simulink model "ABS_Relay_Inf"  (Simulink 6.2)
settings: Solver=ode5  SolverMode=SingleTasking  StartTime=0.0  StopTime=400  FixedStep=0.01  RelTol=1e-3  AbsTol=1e-6
undefined symbols (not defined in the file): ABSPositionScale, ABSPowerScale, ABSTemperatureScale, ABSVelocityScale, mex_baseaddress
libraries: simulink_extras x3, simulink x2
settings Model: Creator=jims  LastModifiedBy=Administrator  ExtModeTrigDuration=40000
settings ConfigSet: SimulationMode=external
settings DataIOCC: ExternalInput=[]  InitialState=[]  LimitDataPoints=off  MaxDataPoints=5000  SaveOutput=off  SaveTime=off  SignalLoggingName=sigsOut
settings OptimizationCC: BlockReduction=off  BooleanDataType=off
settings DebuggingCC: IntegerOverflowMsg=none
settings HardwareCC: TargetEndianess=LittleEndian  TargetHWDeviceType=MATLAB Host
settings RTWCC: SystemTargetFile=rtwin.tlc  TemplateMakefile=rtwin.tmf  Description=Real-Time Windows Target  ProcessScript=rtwin_make_rtw_hook
settings RTWinTargetCC: TargetFcnLib=ansi_tfl_tmw.mat  GenFloatMathFcnCalls=ANSI_C  ModelReferenceCompliant=off  CCOptimize=on

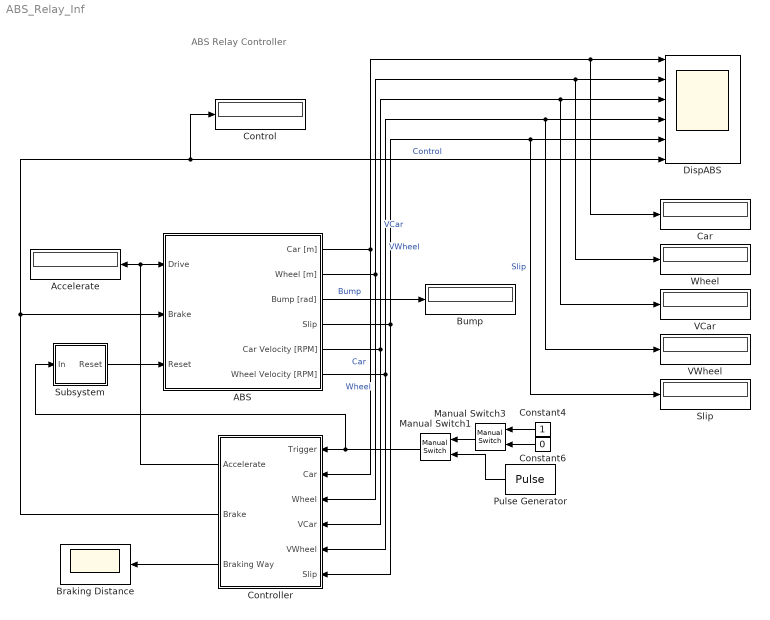
== system ABS_Relay_Inf ==
  note: ABS Relay Controller
  ABS : Subsystem  mask{BaseAddress=mex_baseaddress(-1,-1), T0=0.01}
      mask prompts: BaseAddress "Base Address"; T0 "Sample Time"
      mask Display: image(imread('abs.bmp'))
  Accelerate : Display
  Braking Distance : Scope
      settings: TimeRange=400  YMin=0  YMax=12  SaveName=ABSBrakingDistance  MaxDataPoints=40000
  Bump : Display
  Car : Display
  Constant4 : Constant  Orientation=left
  Constant6 : Constant  Orientation=left  Value=0
  Control : Display
  Controller : Subsystem  Orientation=left
  DispABS : Scope  NumInputPorts=6
      settings: TimeRange=400  YMin=0~0~0~0~-1.5~0  YMax=175~175~2500~2500~2~1  SaveName=ABSHistory  MaxDataPoints=40000
  Manual Switch1 : simulink/Signal Routing/Manual Switch  Orientation=left  sw=0  action=0
  Manual Switch3 : simulink/Signal Routing/Manual Switch  Orientation=left  sw=1  action=0
  Pulse Generator : DiscretePulseGenerator  Orientation=left  PulseType=Time based  Period=20  PulseWidth=90
  Slip : Display
  Subsystem : Subsystem
  VCar : Display
  VWheel : Display
  Wheel : Display
  wires:
  ABS/4(Slip) -> Slip/1, DispABS/5, Controller/6(Slip)  "Slip"
  ABS/6(Wheel Velocity [RPM]) -> VWheel/1, DispABS/4, Controller/5(VWheel)  "VWheel"
  ABS/2(Wheel [m]) -> Wheel/1, DispABS/2, Controller/3(Wheel)  "Wheel"
  ABS/1(Car [m]) -> Car/1, DispABS/1, Controller/2(Car)  "Car"
  Controller/3(Braking Way) -> Braking Distance/1
  Constant6/1 -> Manual Switch3/2
  Constant4/1 -> Manual Switch3/1
  Controller/2(Brake) -> Control/1, DispABS/6, ABS/2(Brake)  "Control"
  ABS/5(Car Velocity [RPM]) -> VCar/1, DispABS/3, Controller/4(VCar)  "VCar"
  ABS/3(Bump [rad]) -> Bump/1  "Bump"
  Controller/1(Accelerate) -> ABS/1(Drive), Accelerate/1
  Manual Switch3/1 -> Manual Switch1/1
  Pulse Generator/1 -> Manual Switch1/2
  Manual Switch1/1 -> Controller/1(Trigger), Subsystem/1(In)
  Subsystem/1(Reset) -> ABS/3(Reset)

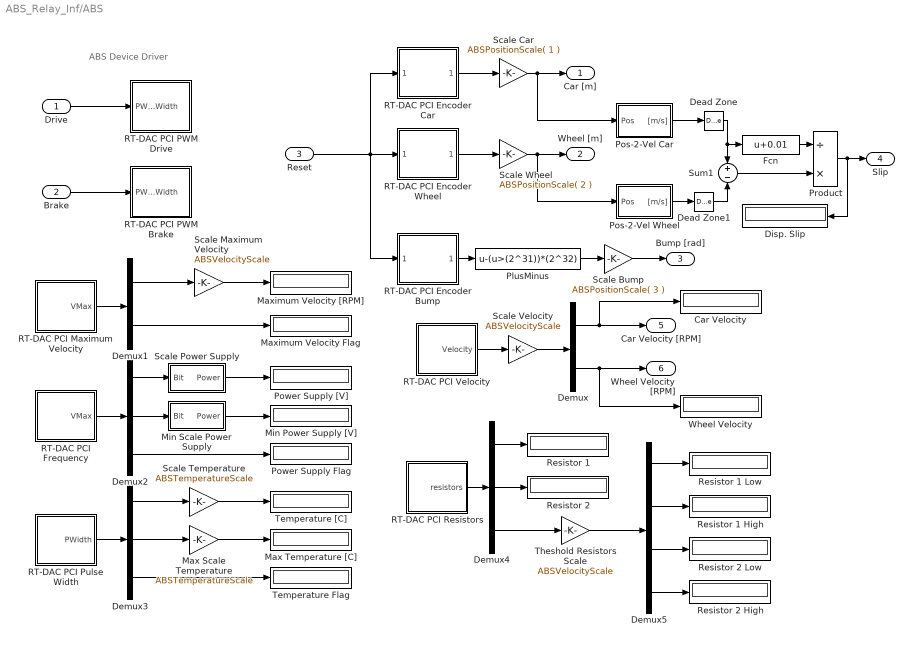
== system ABS_Relay_Inf/ABS ==
  note: ABS Device Driver
  Drive : Inport  Port=1  LatchInput=off
  Brake : Inport  Port=2  LatchInput=off
  Reset : Inport  Port=3  LatchInput=off
  Car Velocity : Display
  Dead Zone : DeadZone  LowerValue=-0.05  UpperValue=0.05  SaturateOnIntegerOverflow=on
  Dead Zone1 : DeadZone  LowerValue=-0.05  UpperValue=0.05  SaturateOnIntegerOverflow=on
  Demux : Demux  Outputs=2
  Demux1 : Demux  Outputs=2
  Demux2 : Demux  Outputs=3
  Demux3 : Demux  Outputs=3
  Demux4 : Demux  Outputs=[1 1 4]
  Demux5 : Demux
  Disp. Slip : Display
      settings: Format=bank
  Fcn : Fcn  Expr=u+0.01
  Max Scale Temperature : Gain  Gain=ABSTemperatureScale
  Max Temperature [C] : Display
  Maximum Velocity Flag : Display
  Maximum Velocity [RPM] : Display
  Min Power Supply [V] : Display
  Min Scale Power Supply : Subsystem
  PlusMinus : Fcn  Expr=u-(u>(2^31))*(2^32)
  Pos-2-Vel Car : Subsystem
  Pos-2-Vel Wheel : Subsystem
  Power Supply Flag : Display
  Power Supply [V] : Display
  Product : Product  Inputs=/*  SaturateOnIntegerOverflow=on  InputSameDT=on
  RT-DAC PCI Encoder Bump : Subsystem  mask(Incremental Encoders){BaseAddress=BaseAddress, ChannelIdx=2, T0=T0}
      mask prompts: BaseAddress "Base Address:"; ChannelIdx "Channel:"; T0 "Sample Time (sec):"
      mask help: RT-DAC PCI Device Driver
      mask Help: Set up each field for your specific hardware configuration.
      mask StyleString: edit,popup(0|1|2|3),edit
      mask Display: plot(0,0,100,100,[90,80,80,11,11],[90,90,20,20,80],[11,80],[80,80],[80,80],[20,14],[80,85,85,80],[45,45,66,66],[45,45,74,74],[20,13,13,20],[15,27,27,15,15],[75,75,26,26,75],[33,48,48,33,33],[75,75,55,55,75],[55,55,71,71,55],[55,75,75,55,55],[33,41,41,33,33],[50,50,27,27,50],[48,56,56,48,48],[50,50,27,27,50],[62,70,70,62,62],[50,50,27,27,50])
  RT-DAC PCI Encoder Car : Subsystem  mask(Incremental Encoders){BaseAddress=BaseAddress, ChannelIdx=0, T0=T0}
      mask prompts: BaseAddress "Base Address:"; ChannelIdx "Channel:"; T0 "Sample Time (sec):"
      mask help: RT-DAC PCI Device Driver
      mask Help: Set up each field for your specific hardware configuration.
      mask StyleString: edit,popup(0|1|2|3),edit
      mask Display: plot(0,0,100,100,[90,80,80,11,11],[90,90,20,20,80],[11,80],[80,80],[80,80],[20,14],[80,85,85,80],[45,45,66,66],[45,45,74,74],[20,13,13,20],[15,27,27,15,15],[75,75,26,26,75],[33,48,48,33,33],[75,75,55,55,75],[55,55,71,71,55],[55,75,75,55,55],[33,41,41,33,33],[50,50,27,27,50],[48,56,56,48,48],[50,50,27,27,50],[62,70,70,62,62],[50,50,27,27,50])
  RT-DAC PCI Encoder Wheel : Subsystem  mask(Incremental Encoders){BaseAddress=BaseAddress, ChannelIdx=1, T0=T0}
      mask prompts: BaseAddress "Base Address:"; ChannelIdx "Channel:"; T0 "Sample Time (sec):"
      mask help: RT-DAC PCI Device Driver
      mask Help: Set up each field for your specific hardware configuration.
      mask StyleString: edit,popup(0|1|2|3),edit
      mask Display: plot(0,0,100,100,[90,80,80,11,11],[90,90,20,20,80],[11,80],[80,80],[80,80],[20,14],[80,85,85,80],[45,45,66,66],[45,45,74,74],[20,13,13,20],[15,27,27,15,15],[75,75,26,26,75],[33,48,48,33,33],[75,75,55,55,75],[55,55,71,71,55],[55,75,75,55,55],[33,41,41,33,33],[50,50,27,27,50],[48,56,56,48,48],[50,50,27,27,50],[62,70,70,62,62],[50,50,27,27,50])
  RT-DAC PCI Frequency : Subsystem  mask(Incremental Encoders){BaseAddress=BaseAddress, T0=T0}
      mask prompts: BaseAddress "Base Address:"; T0 "Sample Time (sec):"
      mask help: RT-DAC PCI Device Driver
      mask Help: Set up each field for your specific hardware configuration.
      mask Display: plot(0,0,100,100,[90,80,80,11,11],[90,90,20,20,80],[11,80],[80,80],[80,80],[20,14],[80,85,85,80],[45,45,66,66],[45,45,74,74],[20,13,13,20],[15,27,27,15,15],[75,75,26,26,75],[33,48,48,33,33],[75,75,55,55,75],[55,55,71,71,55],[55,75,75,55,55],[33,41,41,33,33],[50,50,27,27,50],[48,56,56,48,48],[50,50,27,27,50],[62,70,70,62,62],[50,50,27,27,50])
  RT-DAC PCI Maximum Velocity : Subsystem  mask(Incremental Encoders){BaseAddress=BaseAddress, T0=T0}
      mask prompts: BaseAddress "Base Address:"; T0 "Sample Time (sec):"
      mask help: RT-DAC PCI Device Driver
      mask Help: Set up each field for your specific hardware configuration.
      mask Display: plot(0,0,100,100,[90,80,80,11,11],[90,90,20,20,80],[11,80],[80,80],[80,80],[20,14],[80,85,85,80],[45,45,66,66],[45,45,74,74],[20,13,13,20],[15,27,27,15,15],[75,75,26,26,75],[33,48,48,33,33],[75,75,55,55,75],[55,55,71,71,55],[55,75,75,55,55],[33,41,41,33,33],[50,50,27,27,50],[48,56,56,48,48],[50,50,27,27,50],[62,70,70,62,62],[50,50,27,27,50])
  RT-DAC PCI PWM Brake : Subsystem  mask(PWM Module){BaseAddress=BaseAddress, ChanIdx=1, ChanMode=12 Bit, ChanPresc=60, SetOutputsFlag=on, SetOutputsValue=0, T0=T0}
      mask prompts: BaseAddress "IO Base Address:"; ChanIdx "Channel:"; ChanMode "Channel Mode:"; ChanPresc "Channel Prescaler:"; SetOutputsFlag "Set Outputs At Termination"; SetOutputsValue "Termination Outputs:"; T0 "Sample Time (sec):"
      mask help: RT-DAC PCI Device Driver
      mask Help: Set up each field for your specific hardware configuration.
      mask StyleString: edit,popup(0|1|2|3),popup(8 Bit|12 Bit),edit,checkbox,edit,edit
      mask Display: plot(0,0,100,100,[90,80,80,11,11],[90,90,20,20,80],[11,80],[80,80],[80,80],[20,14],[80,85,85,80],[45,45,66,66],[45,45,74,74],[20,13,13,20],[15,27,27,15,15],[75,75,26,26,75],[33,48,48,33,33],[75,75,55,55,75],[55,55,71,71,55],[55,75,75,55,55],[33,41,41,33,33],[50,50,27,27,50],[48,56,56,48,48],[50,50,27,27,50],[62,70,70,62,62],[50,50,27,27,50])
  RT-DAC PCI PWM Drive : Subsystem  mask(PWM Module){BaseAddress=BaseAddress, ChanIdx=0, ChanMode=12 Bit, ChanPresc=60, SetOutputsFlag=on, SetOutputsValue=0, T0=T0}
      mask prompts: BaseAddress "IO Base Address:"; ChanIdx "Channel:"; ChanMode "Channel Mode:"; ChanPresc "Channel Prescaler:"; SetOutputsFlag "Set Outputs At Termination"; SetOutputsValue "Termination Outputs:"; T0 "Sample Time (sec):"
      mask help: RT-DAC PCI Device Driver
      mask Help: Set up each field for your specific hardware configuration.
      mask StyleString: edit,popup(0|1|2|3),popup(8 Bit|12 Bit),edit,checkbox,edit,edit
      mask Display: plot(0,0,100,100,[90,80,80,11,11],[90,90,20,20,80],[11,80],[80,80],[80,80],[20,14],[80,85,85,80],[45,45,66,66],[45,45,74,74],[20,13,13,20],[15,27,27,15,15],[75,75,26,26,75],[33,48,48,33,33],[75,75,55,55,75],[55,55,71,71,55],[55,75,75,55,55],[33,41,41,33,33],[50,50,27,27,50],[48,56,56,48,48],[50,50,27,27,50],[62,70,70,62,62],[50,50,27,27,50])
  RT-DAC PCI Pulse Width : Subsystem  mask(Incremental Encoders){BaseAddress=BaseAddress, T0=T0}
      mask prompts: BaseAddress "Base Address:"; T0 "Sample Time (sec):"
      mask help: RT-DAC PCI Device Driver
      mask Help: Set up each field for your specific hardware configuration.
      mask Display: plot(0,0,100,100,[90,80,80,11,11],[90,90,20,20,80],[11,80],[80,80],[80,80],[20,14],[80,85,85,80],[45,45,66,66],[45,45,74,74],[20,13,13,20],[15,27,27,15,15],[75,75,26,26,75],[33,48,48,33,33],[75,75,55,55,75],[55,55,71,71,55],[55,75,75,55,55],[33,41,41,33,33],[50,50,27,27,50],[48,56,56,48,48],[50,50,27,27,50],[62,70,70,62,62],[50,50,27,27,50])
  RT-DAC PCI Resistors : Subsystem  mask(Incremental Encoders){BaseAddress=BaseAddress, T0=T0}
      mask prompts: BaseAddress "Base Address:"; T0 "Sample Time (sec):"
      mask help: RT-DAC PCI Device Driver
      mask Help: Set up each field for your specific hardware configuration.
      mask Display: plot(0,0,100,100,[90,80,80,11,11],[90,90,20,20,80],[11,80],[80,80],[80,80],[20,14],[80,85,85,80],[45,45,66,66],[45,45,74,74],[20,13,13,20],[15,27,27,15,15],[75,75,26,26,75],[33,48,48,33,33],[75,75,55,55,75],[55,55,71,71,55],[55,75,75,55,55],[33,41,41,33,33],[50,50,27,27,50],[48,56,56,48,48],[50,50,27,27,50],[62,70,70,62,62],[50,50,27,27,50])
  RT-DAC PCI Velocity : Subsystem  mask(Incremental Encoders){BaseAddress=BaseAddress, T0=T0}
      mask prompts: BaseAddress "Base Address:"; T0 "Sample Time (sec):"
      mask help: RT-DAC PCI Device Driver
      mask Help: Set up each field for your specific hardware configuration.
      mask Display: plot(0,0,100,100,[90,80,80,11,11],[90,90,20,20,80],[11,80],[80,80],[80,80],[20,14],[80,85,85,80],[45,45,66,66],[45,45,74,74],[20,13,13,20],[15,27,27,15,15],[75,75,26,26,75],[33,48,48,33,33],[75,75,55,55,75],[55,55,71,71,55],[55,75,75,55,55],[33,41,41,33,33],[50,50,27,27,50],[48,56,56,48,48],[50,50,27,27,50],[62,70,70,62,62],[50,50,27,27,50])
  Resistor 1 : Display
  Resistor 1 High : Display
  Resistor 1 Low : Display
  Resistor 2 : Display
  Resistor 2 High : Display
  Resistor 2 Low : Display
  Scale Bump : Gain  Gain=ABSPositionScale( 3 )
  Scale Car : Gain  Gain=ABSPositionScale( 1 )
  Scale Maximum Velocity : Gain  Gain=ABSVelocityScale
  Scale Velocity : Gain  Gain=ABSVelocityScale
  Scale Wheel : Gain  Gain=ABSPositionScale( 2 )
  Scale Power Supply : Subsystem
  Scale Temperature : Gain  Gain=ABSTemperatureScale
  Sum1 : Sum  Inputs=+-  SaturateOnIntegerOverflow=on  InputSameDT=on
  Temperature Flag : Display
  Temperature [C] : Display
  Theshold Resistors Scale : Gain  Gain=ABSVelocityScale
  Wheel Velocity : Display
  Car [m] : Outport
  Wheel [m] : Outport  Port=2
  Bump [rad] : Outport  Port=3
  Slip : Outport  Port=4
  Car Velocity [RPM] : Outport  Port=5
  Wheel Velocity [RPM] : Outport  Port=6
  wires:
  Dead Zone1/1 -> Sum1/2
  Dead Zone/1 -> Fcn/1, Sum1/1
  Pos-2-Vel Car/1("[m/s]") -> Dead Zone/1
  Pos-2-Vel Wheel/1("[m/s]") -> Dead Zone1/1
  Product/1 -> Disp. Slip/1, Slip/1
  Fcn/1 -> Product/1
  Sum1/1 -> Product/2
  Demux5/4 -> Resistor 2 High/1
  Demux5/3 -> Resistor 2 Low/1
  Demux5/2 -> Resistor 1 High/1
  Demux5/1 -> Resistor 1 Low/1
  Theshold Resistors Scale/1 -> Demux5/1
  Demux4/3 -> Theshold Resistors Scale/1
  Demux4/2 -> Resistor 2/1
  Demux4/1 -> Resistor 1/1
  RT-DAC PCI Resistors/1(resistors) -> Demux4/1
  Demux3/3 -> Temperature Flag/1
  Demux3/2 -> Max Scale Temperature/1
  Max Scale Temperature/1 -> Max Temperature [C]/1
  Demux2/3 -> Power Supply Flag/1
  Min Scale Power Supply/1(Power) -> Min Power Supply [V]/1
  Demux2/2 -> Min Scale Power Supply/1(Bit)
  Reset/1 -> RT-DAC PCI Encoder Bump/1(Reset), RT-DAC PCI Encoder Car/1(Reset), RT-DAC PCI Encoder Wheel/1(Reset)
  Demux3/1 -> Scale Temperature/1
  RT-DAC PCI Pulse Width/1(PWidth) -> Demux3/1
  Demux2/1 -> Scale Power Supply/1(Bit)
  RT-DAC PCI Frequency/1(VMax) -> Demux2/1
  Demux1/2 -> Maximum Velocity Flag/1
  Scale Maximum Velocity/1 -> Maximum Velocity [RPM]/1
  Demux1/1 -> Scale Maximum Velocity/1
  RT-DAC PCI Maximum Velocity/1(VMax) -> Demux1/1
  Demux/2 -> Wheel Velocity/1, Wheel Velocity [RPM]/1
  Demux/1 -> Car Velocity/1, Car Velocity [RPM]/1
  Brake/1 -> RT-DAC PCI PWM Brake/1(PWM Width)
  Drive/1 -> RT-DAC PCI PWM Drive/1(PWM Width)
  Scale Temperature/1 -> Temperature [C]/1
  Scale Power Supply/1(Power) -> Power Supply [V]/1
  Scale Velocity/1 -> Demux/1
  RT-DAC PCI Velocity/1(Velocity) -> Scale Velocity/1
  Scale Bump/1 -> Bump [rad]/1
  Scale Wheel/1 -> Pos-2-Vel Wheel/1(Pos), Wheel [m]/1
  Scale Car/1 -> Pos-2-Vel Car/1(Pos), Car [m]/1
  RT-DAC PCI Encoder Bump/1(Encoder Counter) -> PlusMinus/1
  RT-DAC PCI Encoder Wheel/1(Encoder Counter) -> Scale Wheel/1
  RT-DAC PCI Encoder Car/1(Encoder Counter) -> Scale Car/1
  PlusMinus/1 -> Scale Bump/1

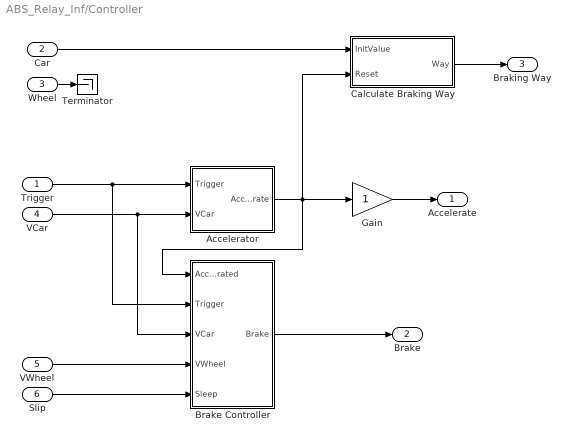
== system ABS_Relay_Inf/Controller ==
  Trigger : Inport  Port=1  LatchInput=off
  Car : Inport  Port=2  LatchInput=off
  Wheel : Inport  Port=3  LatchInput=off
  VCar : Inport  Port=4  LatchInput=off
  VWheel : Inport  Port=5  LatchInput=off
  Slip : Inport  Port=6  LatchInput=off
  Accelerator : Subsystem
  Brake Controller : Subsystem
  Calculate Braking Way : Subsystem
  Gain : Gain  SaturateOnIntegerOverflow=on
  Terminator : Terminator
  Accelerate : Outport
  Brake : Outport  Port=2
  Braking Way : Outport  Port=3
  wires:
  Gain/1 -> Accelerate/1
  Wheel/1 -> Terminator/1
  Brake Controller/1(Brake) -> Brake/1
  VWheel/1 -> Brake Controller/4(VWheel)
  Accelerator/1(Accelerate) -> Gain/1, Brake Controller/1(Accelerated), Calculate Braking Way/2(Reset)
  Slip/1 -> Brake Controller/5(Sleep)
  Car/1 -> Calculate Braking Way/1(InitValue)
  VCar/1 -> Accelerator/2(VCar), Brake Controller/3(VCar)
  Calculate Braking Way/1(Way) -> Braking Way/1
  Trigger/1 -> Brake Controller/2(Trigger), Accelerator/1(Trigger)

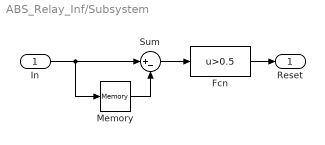
== system ABS_Relay_Inf/Subsystem ==
  In : Inport  Port=1  LatchInput=off
  Fcn : Fcn  Expr=u>0.5
  Memory : Memory
  Sum : Sum  Inputs=|+-  SaturateOnIntegerOverflow=on  InputSameDT=on
  Reset : Outport
  wires:
  Sum/1 -> Fcn/1
  In/1 -> Sum/1, Memory/1
  Fcn/1 -> Reset/1
  Memory/1 -> Sum/2

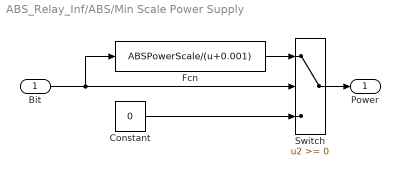
== system ABS_Relay_Inf/ABS/Min Scale Power Supply ==
  Bit : Inport  Port=1  LatchInput=off
  Constant : Constant  Value=0
  Fcn : Fcn  Expr=ABSPowerScale/(u+0.001)
  Switch : Switch  SaturateOnIntegerOverflow=on  InputSameDT=on
  Power : Outport
  wires:
  Bit/1 -> Switch/2, Fcn/1
  Switch/1 -> Power/1
  Fcn/1 -> Switch/1
  Constant/1 -> Switch/3

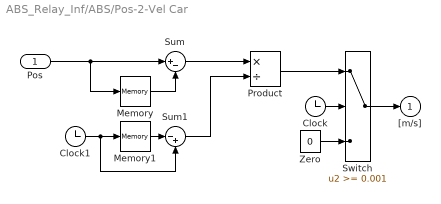
== system ABS_Relay_Inf/ABS/Pos-2-Vel Car ==
  Pos : Inport  Port=1  LatchInput=off
  Clock : Clock
      settings: Decimation=10
  Clock1 : Clock
      settings: Decimation=10
  Memory : Memory  InheritSampleTime=on
  Memory1 : Memory  InheritSampleTime=on
  Product : Product  Inputs=*/  SaturateOnIntegerOverflow=on  InputSameDT=on
  Sum : Sum  Inputs=|+-  SaturateOnIntegerOverflow=on  InputSameDT=on
  Sum1 : Sum  Inputs=|-+  SaturateOnIntegerOverflow=on  InputSameDT=on
  Switch : Switch  Threshold=0.001  SaturateOnIntegerOverflow=on  InputSameDT=on
  Zero : Constant  Value=0
  "[m/s]" : Outport  InitialOutput=0
  wires:
  Pos/1 -> Memory/1, Sum/1
  Memory/1 -> Sum/2
  Clock/1 -> Switch/2
  Switch/1 -> "[m/s]"/1
  Zero/1 -> Switch/3
  Product/1 -> Switch/1
  Sum/1 -> Product/1
  Clock1/1 -> Memory1/1, Sum1/2
  Memory1/1 -> Sum1/1
  Sum1/1 -> Product/2

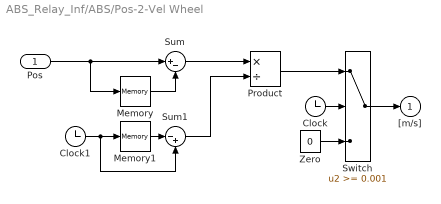
== system ABS_Relay_Inf/ABS/Pos-2-Vel Wheel ==
  Pos : Inport  Port=1  LatchInput=off
  Clock : Clock
      settings: Decimation=10
  Clock1 : Clock
      settings: Decimation=10
  Memory : Memory  InheritSampleTime=on
  Memory1 : Memory  InheritSampleTime=on
  Product : Product  Inputs=*/  SaturateOnIntegerOverflow=on  InputSameDT=on
  Sum : Sum  Inputs=|+-  SaturateOnIntegerOverflow=on  InputSameDT=on
  Sum1 : Sum  Inputs=|-+  SaturateOnIntegerOverflow=on  InputSameDT=on
  Switch : Switch  Threshold=0.001  SaturateOnIntegerOverflow=on  InputSameDT=on
  Zero : Constant  Value=0
  "[m/s]" : Outport  InitialOutput=0
  wires:
  Sum1/1 -> Product/2
  Memory1/1 -> Sum1/1
  Clock1/1 -> Sum1/2, Memory1/1
  Sum/1 -> Product/1
  Product/1 -> Switch/1
  Zero/1 -> Switch/3
  Switch/1 -> "[m/s]"/1
  Clock/1 -> Switch/2
  Memory/1 -> Sum/2
  Pos/1 -> Sum/1, Memory/1

== system ABS_Relay_Inf/ABS/RT-DAC PCI Encoder Bump ==
  Reset : Inport  Port=1  LatchInput=off
  RT-DAC PCI Encoder : S-Function  FunctionName=rtdacpci_abs_encoder  Parameters=BaseAddress, ChannelIdx, T0
  Encoder Counter : Outport  InitialOutput=0
  wires:
  RT-DAC PCI Encoder/1 -> Encoder Counter/1
  Reset/1 -> RT-DAC PCI Encoder/1

== system ABS_Relay_Inf/ABS/RT-DAC PCI Encoder Car ==
  Reset : Inport  Port=1  LatchInput=off
  RT-DAC PCI Encoder : S-Function  FunctionName=rtdacpci_abs_encoder  Parameters=BaseAddress, ChannelIdx, T0
  Encoder Counter : Outport  InitialOutput=0
  wires:
  RT-DAC PCI Encoder/1 -> Encoder Counter/1
  Reset/1 -> RT-DAC PCI Encoder/1

== system ABS_Relay_Inf/ABS/RT-DAC PCI Encoder Wheel ==
  Reset : Inport  Port=1  LatchInput=off
  RT-DAC PCI Encoder : S-Function  FunctionName=rtdacpci_abs_encoder  Parameters=BaseAddress, ChannelIdx, T0
  Encoder Counter : Outport  InitialOutput=0
  wires:
  Reset/1 -> RT-DAC PCI Encoder/1
  RT-DAC PCI Encoder/1 -> Encoder Counter/1

== system ABS_Relay_Inf/ABS/RT-DAC PCI Frequency ==
  RT-DAC PCI Frequency : S-Function  FunctionName=rtdacpci_abs_frequency  Parameters=BaseAddress, T0
  VMax : Outport  InitialOutput=0
  wires:
  RT-DAC PCI Frequency/1 -> VMax/1

== system ABS_Relay_Inf/ABS/RT-DAC PCI Maximum Velocity ==
  RT-DAC PCI VMax : S-Function  FunctionName=rtdacpci_abs_vmax  Parameters=BaseAddress, T0
  VMax : Outport  InitialOutput=0
  wires:
  RT-DAC PCI VMax/1 -> VMax/1

== system ABS_Relay_Inf/ABS/RT-DAC PCI PWM Brake ==
  PWM Width : Inport  Port=1  LatchInput=off
  "RT-DAC PCI PWM " : S-Function  FunctionName=rtdacpci_abs_pwm  Parameters=BaseAddress, ChanIdx, ChanMode, ChanPresc, SetOutputsFlag, SetOutputsValue, T0
  wires:
  PWM Width/1 -> "RT-DAC PCI PWM "/1

== system ABS_Relay_Inf/ABS/RT-DAC PCI PWM Drive ==
  PWM Width : Inport  Port=1  LatchInput=off
  "RT-DAC PCI PWM " : S-Function  FunctionName=rtdacpci_abs_pwm  Parameters=BaseAddress, ChanIdx, ChanMode, ChanPresc, SetOutputsFlag, SetOutputsValue, T0
  wires:
  PWM Width/1 -> "RT-DAC PCI PWM "/1

== system ABS_Relay_Inf/ABS/RT-DAC PCI Pulse Width ==
  RT-DAC PCI Pulse Width : S-Function  FunctionName=rtdacpci_abs_pulsewidth  Parameters=BaseAddress, T0
  PWidth : Outport  InitialOutput=0
  wires:
  RT-DAC PCI Pulse Width/1 -> PWidth/1

== system ABS_Relay_Inf/ABS/RT-DAC PCI Resistors ==
  RT-DAC PCI Resistors : S-Function  FunctionName=rtdacpci_abs_resistors  Parameters=BaseAddress, T0
  resistors : Outport  InitialOutput=0
  wires:
  RT-DAC PCI Resistors/1 -> resistors/1

== system ABS_Relay_Inf/ABS/RT-DAC PCI Velocity ==
  RT-DAC PCI Velocity : S-Function  FunctionName=rtdacpci_abs_velocity  Parameters=BaseAddress, T0
  Velocity : Outport  InitialOutput=0
  wires:
  RT-DAC PCI Velocity/1 -> Velocity/1

== system ABS_Relay_Inf/ABS/Scale Power Supply ==
  Bit : Inport  Port=1  LatchInput=off
  Constant : Constant  Value=0
  Fcn : Fcn  Expr=ABSPowerScale/(u+0.001)
  Switch : Switch  Threshold=0.5  SaturateOnIntegerOverflow=on  InputSameDT=on
  Power : Outport
  wires:
  Constant/1 -> Switch/3
  Fcn/1 -> Switch/1
  Switch/1 -> Power/1
  Bit/1 -> Fcn/1, Switch/2

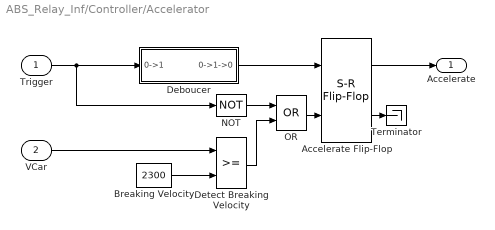
== system ABS_Relay_Inf/Controller/Accelerator ==
  Trigger : Inport  Port=1  LatchInput=off
  VCar : Inport  Port=2  LatchInput=off
  Accelerate Flip-Flop : simulink_extras/Flip Flops/S-R Flip-Flop  initial_condition=0
  Breaking Velocity : Constant  Value=2300
  Deboucer : Subsystem
  Detect Breaking Velocity : RelationalOperator  InputSameDT=on
  NOT : Logic  Operator=NOT
  OR : Logic  Operator=OR
  Terminator : Terminator
  Accelerate : Outport
  wires:
  Accelerate Flip-Flop/1 -> Accelerate/1
  VCar/1 -> Detect Breaking Velocity/1
  Trigger/1 -> NOT/1, Deboucer/1(0->1)
  Accelerate Flip-Flop/2 -> Terminator/1
  NOT/1 -> OR/1
  Detect Breaking Velocity/1 -> OR/2
  OR/1 -> Accelerate Flip-Flop/2
  Breaking Velocity/1 -> Detect Breaking Velocity/2
  Deboucer/1(0->1->0) -> Accelerate Flip-Flop/1

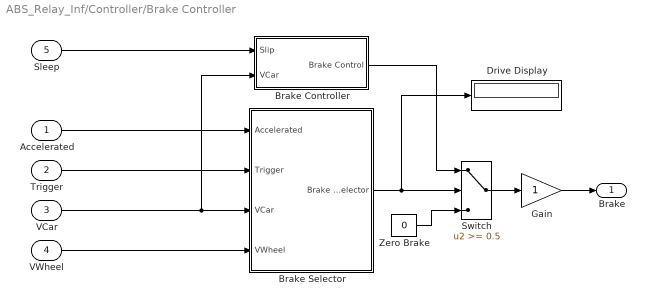
== system ABS_Relay_Inf/Controller/Brake Controller ==
  Accelerated : Inport  Port=1  LatchInput=off
  Trigger : Inport  Port=2  LatchInput=off
  VCar : Inport  Port=3  LatchInput=off
  VWheel : Inport  Port=4  LatchInput=off
  Sleep : Inport  Port=5  LatchInput=off
  Brake Controller : Subsystem
  Brake Selector : Subsystem
  Drive Display : Display
  Gain : Gain  SaturateOnIntegerOverflow=on
  Switch : Switch  Threshold=0.5  InputSameDT=on
  Zero Brake : Constant  Value=0
  Brake : Outport
  wires:
  Gain/1 -> Brake/1
  Brake Controller/1(Brake Control) -> Switch/1
  Sleep/1 -> Brake Controller/1(Slip)
  Zero Brake/1 -> Switch/3
  Brake Selector/1(Brake Selector) -> Drive Display/1, Switch/2
  Switch/1 -> Gain/1
  VWheel/1 -> Brake Selector/4(VWheel)
  VCar/1 -> Brake Controller/2(VCar), Brake Selector/3(VCar)
  Trigger/1 -> Brake Selector/2(Trigger)
  Accelerated/1 -> Brake Selector/1(Accelerated)

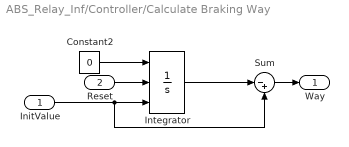
== system ABS_Relay_Inf/Controller/Calculate Braking Way ==
  InitValue : Inport  Port=1  LatchInput=off
  Reset : Inport  Port=2  LatchInput=off
  Constant2 : Constant  Value=0
  Integrator : Integrator  ExternalReset=level  InitialConditionSource=external
  Sum : Sum  Inputs=|-+  SaturateOnIntegerOverflow=on  InputSameDT=on
  Way : Outport
  wires:
  Sum/1 -> Way/1
  Reset/1 -> Integrator/2
  InitValue/1 -> Integrator/3, Sum/2
  Integrator/1 -> Sum/1
  Constant2/1 -> Integrator/1

== system ABS_Relay_Inf/Controller/Accelerator/Deboucer ==
  0->1 : Inport  Port=1  LatchInput=off
  AND : Logic
  Memory : Memory
  NOT : Logic  Operator=NOT
  0->1->0 : Outport
  wires:
  AND/1 -> 0->1->0/1
  0->1/1 -> Memory/1, AND/2
  Memory/1 -> NOT/1
  NOT/1 -> AND/1

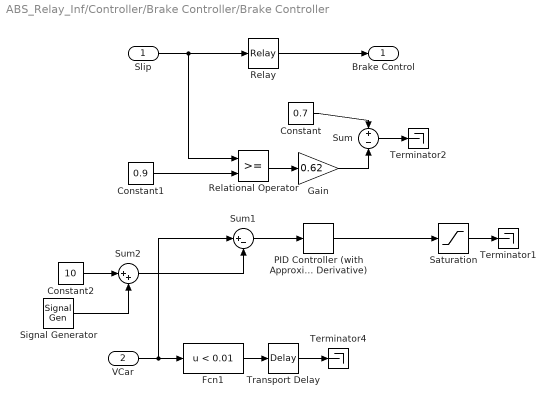
== system ABS_Relay_Inf/Controller/Brake Controller/Brake Controller ==
  Slip : Inport  Port=1  LatchInput=off
  VCar : Inport  Port=2  LatchInput=off
  Constant : Constant  Value=0.7
  Constant1 : Constant  Value=0.9
  Constant2 : Constant  Value=10
  Fcn1 : Fcn  Expr=u < 0.01
  Gain : Gain  Gain=0.62  SaturateOnIntegerOverflow=on
  PID Controller (with Approximate Derivative) : simulink_extras/Additional Linear/PID Controller (with Approximate Derivative)  P=0.2  I=0  D=0  N=100
  Relational Operator : RelationalOperator  InputSameDT=on
  Relay : Relay  OnSwitchValue=0.25  OffSwitchValue=0.1  OnOutputValue=0  OffOutputValue=1
  Saturation : Saturate  UpperLimit=0.7  LowerLimit=0
  Signal Generator : SignalGenerator  WaveForm=square  Amplitude=2  Frequency=0.03
  Sum : Sum  Inputs=+-  SaturateOnIntegerOverflow=on  InputSameDT=on
  Sum1 : Sum  Inputs=|+-  SaturateOnIntegerOverflow=on  InputSameDT=on
  Sum2 : Sum  Inputs=|++  SaturateOnIntegerOverflow=on  InputSameDT=on
  Terminator1 : Terminator
  Terminator2 : Terminator
  Terminator4 : Terminator
  Transport Delay : TransportDelay  DelayTime=0.5
  Brake Control : Outport
  wires:
  Slip/1 -> Relational Operator/1, Relay/1
  Fcn1/1 -> Transport Delay/1
  VCar/1 -> Fcn1/1, Sum1/1
  Relational Operator/1 -> Gain/1
  Constant1/1 -> Relational Operator/2
  Constant/1 -> Sum/1
  Gain/1 -> Sum/2
  Sum1/1 -> PID Controller (with Approximate Derivative)/1
  PID Controller (with Approximate Derivative)/1 -> Saturation/1
  Sum2/1 -> Sum1/2
  Constant2/1 -> Sum2/1
  Signal Generator/1 -> Sum2/2
  Relay/1 -> Brake Control/1
  Sum/1 -> Terminator2/1
  Saturation/1 -> Terminator1/1
  Transport Delay/1 -> Terminator4/1

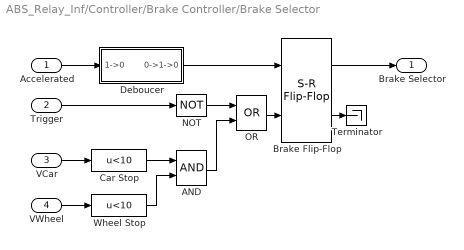
== system ABS_Relay_Inf/Controller/Brake Controller/Brake Selector ==
  Accelerated : Inport  Port=1  LatchInput=off
  Trigger : Inport  Port=2  LatchInput=off
  VCar : Inport  Port=3  LatchInput=off
  VWheel : Inport  Port=4  LatchInput=off
  AND : Logic
  Brake Flip-Flop : simulink_extras/Flip Flops/S-R Flip-Flop  initial_condition=0
  Car Stop : Fcn  Expr=u<10
  Deboucer : Subsystem
  NOT : Logic  Operator=NOT
  OR : Logic  Operator=OR
  Terminator : Terminator
  Wheel Stop : Fcn  Expr=u<10
  Brake Selector : Outport
  wires:
  VWheel/1 -> Wheel Stop/1
  VCar/1 -> Car Stop/1
  Trigger/1 -> NOT/1
  Accelerated/1 -> Deboucer/1(1->0)
  Brake Flip-Flop/1 -> Brake Selector/1
  Wheel Stop/1 -> AND/2
  Car Stop/1 -> AND/1
  Deboucer/1(0->1->0) -> Brake Flip-Flop/1
  OR/1 -> Brake Flip-Flop/2
  AND/1 -> OR/2
  NOT/1 -> OR/1
  Brake Flip-Flop/2 -> Terminator/1

== system ABS_Relay_Inf/Controller/Brake Controller/Brake Selector/Deboucer ==
  1->0 : Inport  Port=1  LatchInput=off
  AND : Logic
  Memory : Memory
  NOT : Logic  Operator=NOT
  0->1->0 : Outport
  wires:
  NOT/1 -> AND/2
  Memory/1 -> AND/1
  1->0/1 -> NOT/1, Memory/1
  AND/1 -> 0->1->0/1
